simulink model "Transfer_fcn"  (R2020a)
settings: Solver=VariableStepAuto  StartTime=0.0  StopTime=10.0  RelTol=1e-3
model workspace (MAT data in the model file):
  B = 1
settings Model: Creator=emami  LastModifiedBy=emami

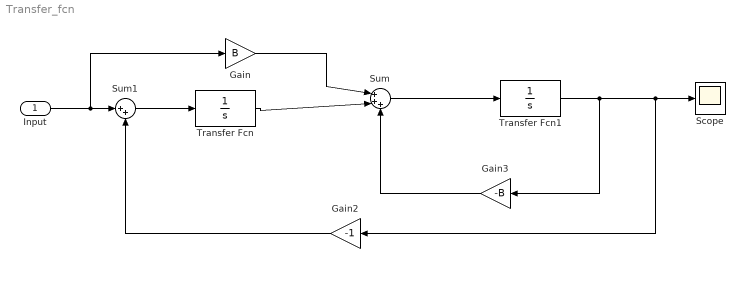
== system Transfer_fcn ==
  Input : Inport
  Gain : Gain  Gain=B
  Gain2 : Gain  Gain=-1
  Gain3 : Gain  Gain=-B
  Scope : Scope
  Sum : Sum  Inputs=|+++
  Sum1 : Sum  Inputs=|++
  Transfer Fcn : TransferFcn  Denominator=[1 0]
  Transfer Fcn1 : TransferFcn  Denominator=[1 0]
  wires:
  Sum/1 -> Transfer Fcn1/1
  Transfer Fcn1/1 -> Gain3/1, Gain2/1, Scope/1
  Gain3/1 -> Sum/3
  Gain/1 -> Sum/1
  Transfer Fcn/1 -> Sum/2
  Gain2/1 -> Sum1/2
  Sum1/1 -> Transfer Fcn/1
  Input/1 -> Gain/1, Sum1/1
